simulink model "PMSM_vector_control_sim"  (R2019a)
settings: Solver=ode4  StartTime=0.0  StopTime=Tfinal  FixedStep=Ts  RelTol=1e-3  EnableMultiTasking=on
values from neighbouring files (symbols this model uses):
  Cdc = 150e-6    (= 0.00015)    [PMSM_modular_vector_control_sim_parameters.m]    (also in PMSM_vector_control_single_parameters.m)
  EfRated = 80    [PMSM_modular_vector_control_sim_parameters.m]    (also in PMSM_vector_control_single_parameters.m)
  fout = 100    [PMSM_modular_vector_control_sim_parameters.m]    (also in PMSM_vector_control_single_parameters.m)
  IdPIDmax = Vdcm/5    (= 20)    [PMSM_modular_vector_control_sim_parameters.m]    (also in PMSM_vector_control_single_parameters.m = 54)
  IdPIDmin = -Vdcm/5    (= -20)    [PMSM_modular_vector_control_sim_parameters.m]    (also in PMSM_vector_control_single_parameters.m = -54)
  Idref = 0    [PMSM_vector_control_single_parameters.m]
  Inertia = 1e-2    (= 0.01)    [PMSM_modular_vector_control_sim_parameters.m]    (also in PMSM_vector_control_single_parameters.m)
  IqPIDmax = Vdcm-10    (= 90)    [PMSM_modular_vector_control_sim_parameters.m]    (also in PMSM_vector_control_single_parameters.m = 260)
  IqPIDmin = -(Vdcm-10)    (= -90)    [PMSM_modular_vector_control_sim_parameters.m]    (also in PMSM_vector_control_single_parameters.m = -260)
  IrefOverTref = MotorSpeedRad/(EfRated*3)    (= 0.261799387799)    [PMSM_modular_vector_control_sim_parameters.m]    (also in PMSM_vector_control_single_parameters.m)
  LoadTorque1 = 2    [PMSM_modular_vector_control_sim_parameters.m]    (also in PMSM_vector_control_single_parameters.m = 30)
  LoadTorque2 = 2    [PMSM_modular_vector_control_sim_parameters.m]    (also in PMSM_vector_control_single_parameters.m = 20)
  LoadTorqueStepTime = 3    [PMSM_modular_vector_control_sim_parameters.m]    (also in PMSM_vector_control_single_parameters.m = 0.5)
  Ls = 3.51e-3    (= 0.00351)    [PMSM_modular_vector_control_sim_parameters.m]    (also in PMSM_vector_control_single_parameters.m)
  modulation_type = 1    [PMSM_modular_vector_control_sim_parameters.m]    (also in PMSM_vector_control_single_parameters.m)
  phase = [0 0 0 0]    [PMSM_modular_vector_control_sim_parameters.m]    (also in PMSM_vector_control_single_parameters.m)
  PolePairs = 10    [PMSM_modular_vector_control_sim_parameters.m]    (also in PMSM_vector_control_single_parameters.m)
  Rin = 1e-3    (= 0.001)    [PMSM_modular_vector_control_sim_parameters.m]    (also in PMSM_vector_control_single_parameters.m)
  Ripth = 0.1    [PMSM_modular_vector_control_sim_parameters.m]    (also in PMSM_vector_control_single_parameters.m)
  Rs = 321e-3    (= 0.321)    [PMSM_modular_vector_control_sim_parameters.m]    (also in PMSM_vector_control_single_parameters.m)
  SpeedPIDmax = 20    [PMSM_modular_vector_control_sim_parameters.m]    (also in PMSM_vector_control_single_parameters.m = 60)
  SpeedPIDmin = -20    [PMSM_modular_vector_control_sim_parameters.m]    (also in PMSM_vector_control_single_parameters.m = -60)
  SpeedRef1 = 200    [PMSM_modular_vector_control_sim_parameters.m]    (also in PMSM_vector_control_single_parameters.m = 600)
  SpeedRef2 = 100    [PMSM_modular_vector_control_sim_parameters.m]    (also in PMSM_vector_control_single_parameters.m = 200)
  SpeedRefStepTime = 6    [PMSM_modular_vector_control_sim_parameters.m]    (also in PMSM_vector_control_single_parameters.m = 0.5)
  Ts = 1000e-9    (= 1e-06)    [PMSM_modular_vector_control_sim_parameters.m]    (also in PMSM_vector_control_single_parameters.m)
  Vdc = 200    [PMSM_modular_vector_control_sim_parameters.m]    (also in PMSM_vector_control_single_parameters.m = 270)
  Vin = Vdc + Rin*(Pout/Vdc)    (= 200.01)    [PMSM_modular_vector_control_sim_parameters.m]    (also in PMSM_vector_control_single_parameters.m = 270.007407407)
  ViscousFriction = 1e-3    (= 0.001)    [PMSM_modular_vector_control_sim_parameters.m]    (also in PMSM_vector_control_single_parameters.m)
undefined symbols (not defined in the file or in its folder): delta, Lload, ma, Rload
libraries: powerlib x28, powerlib_meascontrol x25, simulink x6, electricdrivelib x1
settings Model: Creator=ugurm  LastModifiedBy=hakan
settings DataIOCC: LimitDataPoints=on  SaveFormat=Array  ReturnWorkspaceOutputs=off
settings OptimizationCC: LifeSpan=inf
settings DebuggingCC: UnderspecifiedInitializationDetection=Classic  MergeDetectMultiDrivingBlocksExec=none  SolverPrmCheckMsg=warning  StateNameClashWarn=warning  SFUnexpectedBacktrackingDiag=warning  SFNoUnconditionalDefaultTransitionDiag=warning  ArithmeticOperatorsInVariantConditions=warning
settings HardwareCC: ProdBitPerPointer=32  ProdBitPerSizeT=32  ProdBitPerPtrDiffT=32  ProdLargestAtomicFloat=None  ProdIntDivRoundTo=Undefined  ProdEndianess=Unspecified  ProdWordSize=32  ProdHWDeviceType=32-bit Generic
settings ModelReferenceCC: PropagateSignalLabelsOutOfModel=off
settings SFSimCC: SimUseLocalCustomCode=off
settings RTWCC: RTWUseLocalCustomCode=off
settings CodeAppCC: StateflowObjectComments=on
settings GRTTargetCC: TargetLangStandard=C89/C90 (ANSI)  GeneratePreprocessorConditionals=Disable all
settings ConfigComp: CovMetricSettings=dw  CovHtmlReporting=on  CovSaveCumulativeToWorkspaceVar=on  CovSaveSingleToWorkspaceVar=on  CovExternalEMLEnable=off
settings SimscapeCC: SimscapeNormalizeSystem=off

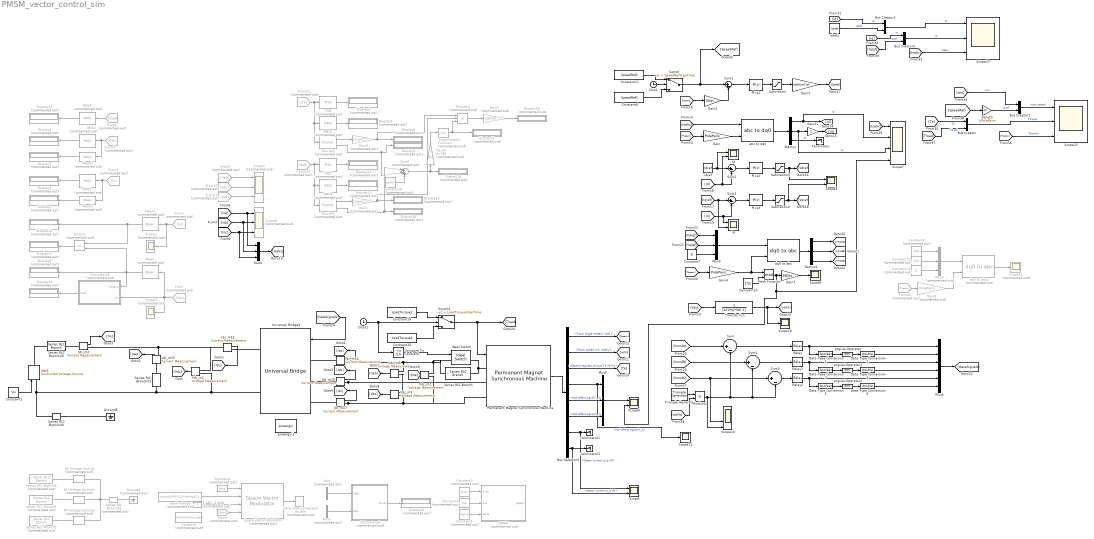
== system PMSM_vector_control_sim ==
  "1:ABC, -1:ACB" : Constant  Commented=on  Value=-1
  AC Voltage Source : powerlib/Electrical Sources/AC Voltage Source  Commented=on  Amplitude=EfRated*sqrt(2)  Phase=0  Frequency=fout  SampleTime=0  Measurements=None  BusType=swing  Pref=10e3  Qref=0  Qmin=-inf  Qmax=+inf
      settings: SourceProductName=Simscape Electrical
  AC Voltage Source1 : powerlib/Electrical Sources/AC Voltage Source  Commented=on  Amplitude=EfRated*sqrt(2)  Phase=-120  Frequency=fout  SampleTime=0  Measurements=None  BusType=swing  Pref=10e3  Qref=0  Qmin=-inf  Qmax=+inf
      settings: SourceProductName=Simscape Electrical
  AC Voltage Source2 : powerlib/Electrical Sources/AC Voltage Source  Commented=on  Amplitude=EfRated*sqrt(2)  Phase=120  Frequency=fout  SampleTime=0  Measurements=None  BusType=swing  Pref=10e3  Qref=0  Qmin=-inf  Qmax=+inf
      settings: SourceProductName=Simscape Electrical
  Bus Creator{,1..3} (4 alike) : BusCreator  Inputs=2
  Bus Selector3 : BusSelector  OutputSignals=Rotor angle thetam (rad),Rotor speed wm (rad/s),Electromagnetic torque Te (N*m),Hall effect signal h_a,Hall effect signal h_b,Hall effect signal h_c,Stator current is_q (A),Stator current is_d (A)
  Clock : Clock
  Clock1 : Clock
  Compare To Constant : simulink/Logic and Bit Operations/Compare To Constant  relop=<=  const=3.0  OutDataTypeStr=boolean
  Constant : Constant  Commented=on  Value=modulation_type
  Constant1 : Constant  Value=Vin
  Constant10 : Constant  Value=2*pi
  Constant11 : Constant  Value=SpeedRef2
  Constant12 : Constant  Commented=on  Value=100
  Constant13 : Constant  Commented=on  Value=0
  Constant14 : Constant  Value=LoadTorque2
  Constant15 : Constant  Value=LoadTorque1
  Constant2 : Constant  Commented=on  Value=fout
  Constant3 : Constant  Commented=on  Value=fout
  Constant4 : Constant  Commented=on  Value=ma
  Constant5 : Constant  Commented=on  Value=delta
  Constant6 : Constant  Value=SpeedRef1
  Constant7 : Constant  Value=0
  Constant8 : Constant  Commented=on  Value=100
  Constant9 : Constant  Commented=on  Value=sqrt(3)
  Data Type Conversion : DataTypeConversion  Commented=on  OutDataTypeStr=double
  Data Type Conversion1 : DataTypeConversion  OutDataTypeStr=boolean
  Data Type Conversion2 : DataTypeConversion  OutDataTypeStr=double
  Data Type Conversion3 : DataTypeConversion  OutDataTypeStr=boolean
  Data Type Conversion4 : DataTypeConversion  OutDataTypeStr=double
  Data Type Conversion5 : DataTypeConversion  OutDataTypeStr=boolean
  Data Type Conversion6 : DataTypeConversion  OutDataTypeStr=double
  Demux : Demux  Outputs=3
  Demux1 : Demux  Outputs=3
  Display{1..21} (21 alike) : Display  Commented=on
  Fourier1 : powerlib_meascontrol/Measurements/Fourier  Commented=on  Freq=fout  n=1  InInit=[0, 0]  Ts=Ts
      settings: SourceProductName=Simscape Electrical
  Fourier2 : powerlib_meascontrol/Measurements/Fourier  Commented=on  Freq=fout  n=1  InInit=[0, 0]  Ts=Ts
      settings: SourceProductName=Simscape Electrical
  From : From  Commented=on  GotoTag=Vdc
  From1 : From  Commented=on  GotoTag=Iin
  From10 : From  Commented=on  GotoTag=Vbc
  From11 : From  Commented=on  GotoTag=Vca
  From12 : From  Commented=on  GotoTag=Isa
  From15 : From  Commented=on  GotoTag=Vab
  From2 : From  Commented=on  GotoTag=Iin
  From3 : From  Commented=on  GotoTag=Idc
  From30 : From  Commented=on  GotoTag=Thetam
  From4 : From  Commented=on  GotoTag=Icap
  From5 : From  Commented=on  GotoTag=Vdc
  From9 : From  Commented=on  GotoTag=Vab
  Gain : Gain  Gain=PolePairs
  Gain1 : Gain  Commented=on  Gain=1/sqrt(2)
  Gain10 : Gain  Gain=1/PolePairs
  Gain11 : Gain
  Gain2 : Gain  Gain=30/pi
  Gain3 : Gain  Gain=IrefOverTref
  Gain4 : Gain  Gain=PolePairs
  Gain5 : Gain  Commented=on  Gain=sqrt(3)
  Gain6 : Gain  Commented=on  Gain=pi/180
  Gain7 : Gain  Gain=180/pi
  Gain8 : Gain  Commented=on  Gain=PolePairs
  Gain9 : Gain  Commented=on  Gain=1/sqrt(2)
  Ground5 : powerlib/Elements/Ground  LConnTagsString=a
      settings: SourceProductName=Simscape Electrical
  Ground6 : powerlib/Elements/Ground  Commented=on  LConnTagsString=a
      settings: SourceProductName=Simscape Electrical
  Id : Scope  NumInputPorts=2
  Idc_m{2,11,14..17} (6 alike) : powerlib/Measurements/Current Measurement  PhasorSimulation=off  OutputType=Complex  PSBequivalent=0
      settings: SourceProductName=Simscape Electrical
  Ideal Switch : powerlib/Power Electronics/Ideal Switch  Ron=0.001  Lon=0  IC=0  Rs=1e5  Cs=inf  Measurements=on
      settings: SourceProductName=Simscape Electrical
  Iq : Scope  NumInputPorts=2
  Logical Operator : Logic  Operator=NOT  AllPortsSameDT=off  OutDataTypeStr=boolean
  Logical Operator1 : Logic  Operator=NOT  AllPortsSameDT=off  OutDataTypeStr=boolean
  Logical Operator2 : Logic  Operator=NOT  AllPortsSameDT=off  OutDataTypeStr=boolean
  Math Function : Math  Operator=mod  SaturateOnIntegerOverflow=on
  Mean{,1..3} (4 alike) : powerlib_meascontrol/Measurements/Mean  Commented=on  Freq=fout  Vinit=0  Ts=0
      settings: SourceProductName=Simscape Electrical
  Mux : Mux  Commented=on  Inputs=3
  Mux1 : Mux  Commented=on  Inputs=3
  Mux2 : Mux  Inputs=3
  Mux3 : Mux  Inputs=3
  Mux4 : Mux  Inputs=6
  Mux5 : Mux  Inputs=3
  Mux6 : Mux  Commented=on  Inputs=3
  PI iq1 : simulink/Continuous/PID Controller  Controller=PI  Form=Parallel  TimeDomain=Discrete-time  SampleTime=-1  IntegratorMethod=Forward Euler  FilterMethod=Forward Euler  ControllerParametersSource=internal  P=0.1  I=1  D=0  UseFilter=on  N=100  TunerSelectOption=Transfer Function Based (PID Tuner App)  InitialConditionSource=internal  InitialConditionForIntegrator=0  InitialConditionForFilter=0  DifferentiatorICPrevScaledInput=0  ExternalReset=none  TrackingMode=off  Kt=1  LimitOutput=off  UpperSaturationLimit=inf  LowerSaturationLimit=-inf  LinearizeAsGain=on  AntiWindupMode=none  Kb=1  POutMin=[]  POutMax=[]  IOutMin=[]  IOutMax=[]  DOutMin=[]  DOutMax=[]  NOutMin=[]  NOutMax=[]  SumOutMin=[]  SumOutMax=[]  SaturationOutMin=[]  SaturationOutMax=[]  PParamMin=[]  PParamMax=[]  IParamMin=[]  IParamMax=[]  DParamMin=[]  DParamMax=[]  NParamMin=[]  NParamMax=[]  KbParamMin=[]  KbParamMax=[]  KtParamMin=[]  KtParamMax=[]  KbOutMin=[]  KbOutMax=[]  KtOutMin=[]  KtOutMax=[]  IntegratorOutMin=[]  IntegratorOutMax=[]  FilterOutMin=[]  FilterOutMax=[]  SumI1OutMin=[]  SumI1OutMax=[]  SumI2OutMin=[]  SumI2OutMax=[]  SumI3OutMin=[]  SumI3OutMax=[]  SumI4OutMin=[]  SumI4OutMax=[]  SumDOutMin=[]  SumDOutMax=[]  DifferentiatorOutMin=[]  DifferentiatorOutMax=[]  FilterDiffOutCoefMin=[]  FilterDiffOutCoefMax=[]  ReciprocalOutMin=[]  ReciprocalOutMax=[]  SumDenOutMin=[]  SumDenOutMax=[]  SumNumOutMin=[]  SumNumOutMax=[]  DivideOutMin=[]  DivideOutMax=[]  IntegratorContinuousStateAttributes=''  IntegratorStateMustResolveToSignalObject=off  IntegratorRTWStateStorageClass=Auto  FilterContinuousStateAttributes=''  FilterStateMustResolveToSignalObject=off  FilterRTWStateStorageClass=Auto  ParallelPVariant=InternalParameters  IdealPVariant=Disabled  IVariant=InternalParameters  DVariant=Disabled  IntegratorVariant=Discrete  SatVariant=Disabled  AWVariant=Passthrough  PCopyVariant=Disabled  TRVariant=Disabled  FdbkBlocksVariant=Forward  IdealPFdbkVariant=Disabled  SatFdbkVariant=Disabled  DerivativeFilterVariant=Disabled  NVariant=Disabled  NCopyVariant=Disabled_SignalSpec  FilterICVariant=Disabled  IntegratorICVariant=InternalICs  ExternalResetVariant=Disabled  TRSumVariant=Passthrough  SumFdbkVariant=Disabled  SumVariant=Sum_PI
  PI iq2 : simulink/Continuous/PID Controller  Controller=PI  Form=Parallel  TimeDomain=Discrete-time  SampleTime=-1  IntegratorMethod=Forward Euler  FilterMethod=Forward Euler  ControllerParametersSource=internal  P=100  I=100  D=0  UseFilter=on  N=100  TunerSelectOption=Transfer Function Based (PID Tuner App)  InitialConditionSource=internal  InitialConditionForIntegrator=0  InitialConditionForFilter=0  DifferentiatorICPrevScaledInput=0  ExternalReset=none  TrackingMode=off  Kt=1  LimitOutput=off  UpperSaturationLimit=inf  LowerSaturationLimit=-inf  LinearizeAsGain=on  AntiWindupMode=none  Kb=1  POutMin=[]  POutMax=[]  IOutMin=[]  IOutMax=[]  DOutMin=[]  DOutMax=[]  NOutMin=[]  NOutMax=[]  SumOutMin=[]  SumOutMax=[]  SaturationOutMin=[]  SaturationOutMax=[]  PParamMin=[]  PParamMax=[]  IParamMin=[]  IParamMax=[]  DParamMin=[]  DParamMax=[]  NParamMin=[]  NParamMax=[]  KbParamMin=[]  KbParamMax=[]  KtParamMin=[]  KtParamMax=[]  KbOutMin=[]  KbOutMax=[]  KtOutMin=[]  KtOutMax=[]  IntegratorOutMin=[]  IntegratorOutMax=[]  FilterOutMin=[]  FilterOutMax=[]  SumI1OutMin=[]  SumI1OutMax=[]  SumI2OutMin=[]  SumI2OutMax=[]  SumI3OutMin=[]  SumI3OutMax=[]  SumI4OutMin=[]  SumI4OutMax=[]  SumDOutMin=[]  SumDOutMax=[]  DifferentiatorOutMin=[]  DifferentiatorOutMax=[]  FilterDiffOutCoefMin=[]  FilterDiffOutCoefMax=[]  ReciprocalOutMin=[]  ReciprocalOutMax=[]  SumDenOutMin=[]  SumDenOutMax=[]  SumNumOutMin=[]  SumNumOutMax=[]  DivideOutMin=[]  DivideOutMax=[]  IntegratorContinuousStateAttributes=''  IntegratorStateMustResolveToSignalObject=off  IntegratorRTWStateStorageClass=Auto  FilterContinuousStateAttributes=''  FilterStateMustResolveToSignalObject=off  FilterRTWStateStorageClass=Auto  ParallelPVariant=InternalParameters  IdealPVariant=Disabled  IVariant=InternalParameters  DVariant=Disabled  IntegratorVariant=Discrete  SatVariant=Disabled  AWVariant=Passthrough  PCopyVariant=Disabled  TRVariant=Disabled  FdbkBlocksVariant=Forward  IdealPFdbkVariant=Disabled  SatFdbkVariant=Disabled  DerivativeFilterVariant=Disabled  NVariant=Disabled  NCopyVariant=Disabled_SignalSpec  FilterICVariant=Disabled  IntegratorICVariant=InternalICs  ExternalResetVariant=Disabled  TRSumVariant=Passthrough  SumFdbkVariant=Disabled  SumVariant=Sum_PI
  PI iq3 : simulink/Continuous/PID Controller  Controller=PI  Form=Parallel  TimeDomain=Discrete-time  SampleTime=-1  IntegratorMethod=Forward Euler  FilterMethod=Forward Euler  ControllerParametersSource=internal  P=100  I=100  D=0  UseFilter=on  N=100  TunerSelectOption=Transfer Function Based (PID Tuner App)  InitialConditionSource=internal  InitialConditionForIntegrator=0  InitialConditionForFilter=0  DifferentiatorICPrevScaledInput=0  ExternalReset=none  TrackingMode=off  Kt=1  LimitOutput=off  UpperSaturationLimit=inf  LowerSaturationLimit=-inf  LinearizeAsGain=on  AntiWindupMode=none  Kb=1  POutMin=[]  POutMax=[]  IOutMin=[]  IOutMax=[]  DOutMin=[]  DOutMax=[]  NOutMin=[]  NOutMax=[]  SumOutMin=[]  SumOutMax=[]  SaturationOutMin=[]  SaturationOutMax=[]  PParamMin=[]  PParamMax=[]  IParamMin=[]  IParamMax=[]  DParamMin=[]  DParamMax=[]  NParamMin=[]  NParamMax=[]  KbParamMin=[]  KbParamMax=[]  KtParamMin=[]  KtParamMax=[]  KbOutMin=[]  KbOutMax=[]  KtOutMin=[]  KtOutMax=[]  IntegratorOutMin=[]  IntegratorOutMax=[]  FilterOutMin=[]  FilterOutMax=[]  SumI1OutMin=[]  SumI1OutMax=[]  SumI2OutMin=[]  SumI2OutMax=[]  SumI3OutMin=[]  SumI3OutMax=[]  SumI4OutMin=[]  SumI4OutMax=[]  SumDOutMin=[]  SumDOutMax=[]  DifferentiatorOutMin=[]  DifferentiatorOutMax=[]  FilterDiffOutCoefMin=[]  FilterDiffOutCoefMax=[]  ReciprocalOutMin=[]  ReciprocalOutMax=[]  SumDenOutMin=[]  SumDenOutMax=[]  SumNumOutMin=[]  SumNumOutMax=[]  DivideOutMin=[]  DivideOutMax=[]  IntegratorContinuousStateAttributes=''  IntegratorStateMustResolveToSignalObject=off  IntegratorRTWStateStorageClass=Auto  FilterContinuousStateAttributes=''  FilterStateMustResolveToSignalObject=off  FilterRTWStateStorageClass=Auto  ParallelPVariant=InternalParameters  IdealPVariant=Disabled  IVariant=InternalParameters  DVariant=Disabled  IntegratorVariant=Discrete  SatVariant=Disabled  AWVariant=Passthrough  PCopyVariant=Disabled  TRVariant=Disabled  FdbkBlocksVariant=Forward  IdealPFdbkVariant=Disabled  SatFdbkVariant=Disabled  DerivativeFilterVariant=Disabled  NVariant=Disabled  NCopyVariant=Disabled_SignalSpec  FilterICVariant=Disabled  IntegratorICVariant=InternalICs  ExternalResetVariant=Disabled  TRSumVariant=Passthrough  SumFdbkVariant=Disabled  SumVariant=Sum_PI
  Permanent Magnet Synchronous Machine : powerlib/Machines/Permanent Magnet Synchronous Machine  NbPhases=3  FluxDistribution=Sinusoidal  RotorType=Round  MechanicalLoad=Torque Tm  PresetModel=No  ShowDetailedParameters=on  MeasurementBus=off  Resistance=Rs  Inductance=8.5e-3  dqInductances=[3.1e-3,3.6e-3]  La=Ls  MachineConstant=Voltage Constant (V_peak L-L / krpm)  Flux=0.18006  VoltageCst=VoltageConstant  TorqueCst=2.7009  Flat=120  Mechanical=[Inertia ViscousFriction PolePairs 0]  PolePairs=4  InitialConditions=[0,0, 0,0]  InitialConditions5ph=[0 0 0 0 0 0]  TsPowergui=0  TsBlock=-1  RefAngle=90 degrees behind phase A axis (modified Park)
  Product : Product  Commented=on
  Product1 : Product
  Product2 : Product  Commented=on  Inputs=3
  RMS{1..5} (5 alike) : powerlib_meascontrol/Measurements/RMS  Commented=on  TrueRMS=on  Freq=fout  RMSInit=0  Ts=0
      settings: SourceProductName=Simscape Electrical
  Relay : Relay
  Relay1 : Relay
  Relay2 : Relay
  SPWM : Subsystem  Commented=on
  Saturation : Saturate  UpperLimit=SpeedPIDmax  LowerLimit=SpeedPIDmin
  Saturation1 : Saturate  UpperLimit=IdPIDmax  LowerLimit=IdPIDmin
  Saturation2 : Saturate  UpperLimit=IqPIDmax  LowerLimit=IqPIDmin
  Scope : Scope  NumInputPorts=2
  Scope1 : Scope  Commented=on
  Scope10 : Scope  NumInputPorts=4
  Scope11 : Scope
  Scope12 : Scope  Commented=on
  Scope13 : Scope  NumInputPorts=3
  Scope15 : Scope  NumInputPorts=3
  Scope16 : Scope
  Scope2 : Scope  Commented=on  NumInputPorts=3
  Scope3 : Scope  Commented=on
  Scope5 : Scope  NumInputPorts=2
  Scope6 : Scope
  Scope7 : Scope  NumInputPorts=4
  Scope8 : Scope  Commented=on  NumInputPorts=3
  Scope9 : Scope  NumInputPorts=2
  Series RLC Branch : powerlib/Elements/Series RLC Branch  LConnTagsString=__new0  RConnTagsString=__new0  BranchType=R  Resistance=5000  Inductance=1e-3  SetiL0=off  InitialCurrent=0  Capacitance=1e-6  Setx0=off  InitialVoltage=0  Measurements=None
      settings: SourceProductName=Simscape Electrical
  Series RLC Branch1 : powerlib/Elements/Series RLC Branch  Commented=on  LConnTagsString=__new0  RConnTagsString=__new0  BranchType=RL  Resistance=Rs  Inductance=Ls  SetiL0=off  InitialCurrent=0  Capacitance=1e-6  Setx0=off  InitialVoltage=0  Measurements=None
      settings: SourceProductName=Simscape Electrical
  Series RLC Branch2 : powerlib/Elements/Series RLC Branch  Commented=on  LConnTagsString=__new0  RConnTagsString=__new0  BranchType=RL  Resistance=Rs  Inductance=Ls  SetiL0=off  InitialCurrent=0  Capacitance=1e-6  Setx0=off  InitialVoltage=0  Measurements=None
      settings: SourceProductName=Simscape Electrical
  Series RLC Branch20 : powerlib/Elements/Series RLC Branch  LConnTagsString=__new0  RConnTagsString=__new0  BranchType=R  Resistance=Rin  Inductance=1e-3  SetiL0=off  InitialCurrent=0  Capacitance=1e-6  Setx0=off  InitialVoltage=0  Measurements=None
      settings: SourceProductName=Simscape Electrical
  Series RLC Branch21 : powerlib/Elements/Series RLC Branch  LConnTagsString=__new0  RConnTagsString=__new0  BranchType=C  Resistance=Rload  Inductance=Lload  SetiL0=off  InitialCurrent=0  Capacitance=Cdc  Setx0=off  InitialVoltage=0  Measurements=None
      settings: SourceProductName=Simscape Electrical
  Series RLC Branch40 : powerlib/Elements/Series RLC Branch  LConnTagsString=__new0  RConnTagsString=__new0  BranchType=R  Resistance=1e12  Inductance=Lload  SetiL0=off  InitialCurrent=0  Capacitance=1e-6  Setx0=off  InitialVoltage=0  Measurements=None
      settings: SourceProductName=Simscape Electrical
  Series RLC Branch42 : powerlib/Elements/Series RLC Branch  Commented=on  LConnTagsString=__new0  RConnTagsString=__new0  BranchType=R  Resistance=1e12  Inductance=Lload  SetiL0=off  InitialCurrent=0  Capacitance=1e-6  Setx0=off  InitialVoltage=0  Measurements=None
      settings: SourceProductName=Simscape Electrical
  Series RLC Branch6 : powerlib/Elements/Series RLC Branch  Commented=on  LConnTagsString=__new0  RConnTagsString=__new0  BranchType=RL  Resistance=Rs  Inductance=Ls  SetiL0=off  InitialCurrent=0  Capacitance=1e-6  Setx0=off  InitialVoltage=0  Measurements=None
      settings: SourceProductName=Simscape Electrical
  Space Vector Modulator : electricdrivelib/Fundamental Drive Blocks/Space Vector Modulator  Commented=on  LabelModeActiveChoice=Detailed  detailLevel=Detailed  fc_bus=50  car_freq=fsw  TsMLIV=1e-6  Ts=Ts
      settings: AttributesFormatString=%<BlockChoice>  SourceProductName=Simscape Electrical  SourceProductBaseCode=PS
  Subsystem4 : Subsystem  Commented=on
  Subsystem5 : Subsystem  Commented=on
  Sum{,1..5} (6 alike) : Sum  Inputs=|+-
  Sum6 : Sum  Commented=on  Inputs=|+--
  Switch : Switch  Criteria=u2 > Threshold  Threshold=SpeedRefStepTime
  Switch1 : Switch  Criteria=u2 > Threshold  Threshold=LoadTorqueStepTime
  THD : powerlib_meascontrol/Measurements/THD  Commented=on  Freq=50  Ts=0
      settings: SourceProductName=Simscape Electrical
  THD1 : powerlib_meascontrol/Measurements/THD  Commented=on  Freq=50  Ts=0
      settings: SourceProductName=Simscape Electrical
  Terminator : Terminator
  Terminator1 : Terminator
  Terminator2 : Terminator
  Transfer Fcn : TransferFcn  Denominator=[1/(2*pi*50) 1]
  Triangle Generator : powerlib_meascontrol/Pulse & Signal Generators/Triangle Generator  Freq=fsw  Phase=phase(1)  Ts=Ts
      settings: SourceProductName=Simscape Electrical
  Trigonometric Function : Trigonometry  Commented=on  Operator=cos
  Universal Bridge4 : powerlib/Power Electronics/Universal Bridge  Arms=3  SnubberResistance=1e5  SnubberCapacitance=inf  Device=IGBT / Diodes  Ron=1e-6  Lon=0  ForwardVoltages="[  0  0  ]"  ForwardVoltage=0  GTOparameters=[ 10e-6 , 20e-6 ]  IGBTparameters=[0,0]  Measurements=None  Measurements_2=None  converterType=Rectifier
      settings: SourceProductName=Simscape Electrical
  Vdc1 : powerlib/Electrical Sources/Controlled Voltage Source  Initialize=off  Source_Type=DC  Amplitude=200  Phase=0  Frequency=0  Measurements=None
      settings: SourceProductName=Simscape Electrical
  Vdc_m{1..3,5} (4 alike) : powerlib/Measurements/Voltage Measurement  PhasorSimulation=off  OutputType=Complex  PSBequivalent=0
      settings: SourceProductName=Simscape Electrical
  abc to dq0 : powerlib_meascontrol/Transformations/abc to dq0  Alignment=90 degrees behind phase A axis
      settings: SourceProductName=Simscape Electrical
  dq0 to abc : powerlib_meascontrol/Transformations/dq0 to abc  Alignment=90 degrees behind phase A axis
      settings: SourceProductName=Simscape Electrical
  dq0 to abc1 : powerlib_meascontrol/Transformations/dq0 to abc  Commented=on  Alignment=Aligned with phase A axis
      settings: SourceProductName=Simscape Electrical
  idref : Constant  Value=Idref
  idref1 : Constant  Value=Idref
  peak voltage : Constant  Commented=on  Value=ma/sqrt(3)*0.612*Vdc*sqrt(2)
  powergui1 : powerlib/powergui  Priority=1  SimulationMode=Discrete  SampleTime=Ts  frequency=60  Iterations=50  frequencyindice=0  Pbase=100e6  ErrMax=1e-4  UnitsV=kV  UnitsW=MW  buscounter=0  FunctionMessages=off  echomessages=off  EnableUseOfTLC=off  CurrentSourceSwitches=off  DisableSnubberDevices=off  DisableRonSwitches=off  DisableVfSwitches=off  DisplayEquations=off  AutomaticDiscreteSolvers=off  SolverType=Tustin  Interpol=off  ExternalGateDelay=off  methode=off  Ts=0  x0status=blocks  SPID=off  SwTol=0  HookPort=off  NonlinearTolerance=0  nMaxIteration=15  ContinueOnMaxIteration=off  RestoreLinks=warning  ResistiveCurrentMeasurement=off  Frange=[0:2:500]  Ylog=off  Xlog=on  ShowGrid=off  save=off  variable=ZData  structure=Icap  ZoomFFT=off  StartTime=0.04  cycles=5  DisplayStyle=3  fundamental=150  FreqAxis=off  MaxFrequency=1000  frequencyindicesteady=1  RmsSteady=1  display=off
      settings: SourceProductName=Simscape Electrical
  wires:
  Idc_m14/1 -> [Isa]
  Constant1/1 -> Vdc1/1
  Idc_m15/1 -> [Icap]
  Idc_m16/1 -> [Isb]
  Idc_m17/1 -> [Isc]
  Mean/1 -> Product/2, Subsystem5/1(Vdcavg), Display8/1
  RMS2/1 -> Display4/1
  Idc_m11/1 -> [Idc]
  Mean3/1 -> Display7/1
  Subsystem5/1(Out1) -> Display14/1
  Product/1 -> Display17/1
  Mux/1 -> Subsystem4/1(Vabc)
  Mux1/1 -> Subsystem4/2(Iabc)
  Subsystem4/1(Poutp) -> Display20/1
  From/1 -> Scope3/1, Mean/1, Subsystem5/2(vdc)
  Mean1/1 -> Display1/1
  RMS1/1 -> Display2/1
  Fourier1/1 -> Gain9/1
  THD/1 -> Display3/1
  RMS4/1 -> Display5/1
  Gain9/1 -> Product2/1, Display6/1
  Fourier1/2 -> Sum6/2, Display9/1
  Vdc_m1/1 -> [Vdc]
  Idc_m2/1 -> [Iin]
  Mean2/1 -> Product/1, Display10/1
  From1/1 -> Scope1/1, Mean2/1
  From2/1 -> Mean1/1, RMS1/1
  From3/1 -> Mean3/1, RMS2/1
  From4/1 -> RMS5/1
  RMS5/1 -> Display11/1
  Constant2/1 -> Space Vector Modulator/1
  From5/1 -> Space Vector Modulator/4
  "1:ABC, -1:ACB"/1 -> Space Vector Modulator/3
  peak voltage/1 -> Space Vector Modulator/2
  Vdc_m5/1 -> [Vab]
  Vdc_m3/1 -> [Vbc]
  Vdc_m2/1 -> [Vca]
  [Isa] -> Mux2/1, Scope8/1
  [Isb] -> Mux2/2, Scope8/2
  [Isc] -> Mux2/3, Scope8/3
  From9/1 -> Scope2/1
  From10/1 -> Scope2/2
  From11/1 -> Scope2/3
  From12/1 -> Fourier1/1, RMS4/1, THD/1
  THD1/1 -> Display12/1
  RMS3/1 -> Display13/1
  From15/1 -> Fourier2/1, RMS3/1, THD1/1
  Space Vector Modulator/1 -> Data Type Conversion/1
  Constant3/1 -> SPWM/1(Freq)
  Constant4/1 -> SPWM/2(ma)
  Constant5/1 -> SPWM/3(delta)
  Permanent Magnet Synchronous Machine/1 -> Bus Selector3/1
  Bus Selector3/3 -> [Te]  "<Electromagnetic torque Te (N*m)>"
  Bus Selector3/2 -> [wm]  "<Rotor speed wm (rad/s)>"
  Bus Selector3/1 -> [Thetam]  "<Rotor angle thetam (rad)>"
  Mux2/1 -> [Isabc]
  [Isabc] -> abc to dq0/1
  Gain/1 -> abc to dq0/2
  [Thetam] -> Gain/1
  abc to dq0/1 -> Demux/1
  Demux/1 -> [id], Scope7/2  "id"
  Demux/2 -> Gain11/1, Scope7/3  "iq"
  Demux/3 -> Terminator/1  "i0"
  Fourier2/1 -> Gain1/1
  Gain1/1 -> Product2/2, Display15/1
  Fourier2/2 -> Sum6/1, Display16/1
  [wm] -> Gain2/1
  Gain2/1 -> Sum1/2
  Switch/1 -> [SpeedRef], Sum1/1
  Sum1/1 -> PI iq1/1
  PI iq1/1 -> Saturation/1
  Saturation/1 -> Gain3/1
  Gain3/1 -> [Iqref]
  [id] -> Id/2, Sum2/2
  Sum2/1 -> PI iq2/1
  PI iq2/1 -> Saturation1/1
  idref/1 -> Id/1, Sum2/1
  [iq] -> Iq/1, Sum3/2
  Sum3/1 -> PI iq3/1
  PI iq3/1 -> Saturation2/1
  [Iqref] -> Iq/2, Sum3/1
  Saturation2/1 -> [Vqref], Scope9/2
  [Thetam] -> Gain4/1
  Gain4/1 -> Math Function/1, dq0 to abc/2
  Constant7/1 -> Mux3/3
  Mux3/1 -> dq0 to abc/1
  [Vdc] -> Transfer Fcn/1
  Transfer Fcn/1 -> Scope16/1, [VdcFilt]
  dq0 to abc/1 -> Demux1/1
  Sum/1 -> Relay/1
  Sum4/1 -> Relay1/1
  Sum5/1 -> Relay2/1
  Data Type Conversion1/1 -> Logical Operator/1
  Logical Operator/1 -> Data Type Conversion2/1
  Data Type Conversion2/1 -> Mux4/2
  Data Type Conversion3/1 -> Logical Operator1/1
  Relay1/1 -> Data Type Conversion3/1, Mux4/3
  Logical Operator1/1 -> Data Type Conversion4/1
  Data Type Conversion4/1 -> Mux4/4
  Data Type Conversion5/1 -> Logical Operator2/1
  Relay2/1 -> Data Type Conversion5/1, Mux4/5
  Logical Operator2/1 -> Data Type Conversion6/1
  Data Type Conversion6/1 -> Mux4/6
  Relay/1 -> Mux4/1, Data Type Conversion1/1
  [VmodC] -> Scope10/3, Sum5/1
  Triangle Generator/1 -> Product1/1
  [VdcFilt] -> Product1/2
  Demux1/1 -> [VmodA]
  Demux1/2 -> [VmodB]
  Demux1/3 -> [VmodC]
  Mux4/1 -> [GateSignals]
  Switch1/1 -> [Tload], Permanent Magnet Synchronous Machine/1
  [GateSignals] -> Universal Bridge4/1
  Product1/1 -> Scope10/4, Sum/2, Sum4/2, Sum5/2
  Constant9/1 -> Sum6/3
  Sum6/1 -> Display18/1, Gain6/1
  Trigonometric Function/1 -> Display21/1, Product2/3
  Gain6/1 -> Trigonometric Function/1
  Product2/1 -> Gain5/1
  Gain5/1 -> Display19/1
  Bus Selector3/6 -> Mux5/3  "<Hall effect signal h_c>"
  Bus Selector3/5 -> Mux5/2  "<Hall effect signal h_b>"
  Bus Selector3/4 -> Scope11/1, Mux5/1  "<Hall effect signal h_a>"
  Mux5/1 -> Scope5/1
  Constant10/1 -> Math Function/2
  Math Function/1 -> Scope7/4, Scope5/2, Gain7/1
  Gain7/1 -> Scope6/1
  [Isabc] -> Scope7/1
  Gain11/1 -> [iq]
  Bus Selector3/7 -> Scope/1, Terminator1/1  "<Stator current is_q (A)>"
  Bus Selector3/8 -> Scope/2, Terminator2/1  "<Stator current is_d (A)>"
  Saturation1/1 -> [Vdref], Scope9/1
  [Vqref] -> Mux3/2
  [Vdref] -> Mux3/1
  Clock/1 -> Switch/2
  Constant11/1 -> Switch/1
  Constant6/1 -> Switch/3
  Clock1/1 -> Compare To Constant/1, Switch1/2
  Constant14/1 -> Switch1/1
  Constant15/1 -> Switch1/3
  Mux6/1 -> dq0 to abc1/1
  Constant8/1 -> Mux6/1
  Constant12/1 -> Mux6/2
  Constant13/1 -> Mux6/3
  From30/1 -> Gain8/1
  Gain8/1 -> dq0 to abc1/2
  dq0 to abc1/1 -> Scope12/1
  [VmodA] -> Sum/1
  [VmodB] -> Sum4/1
  Bus Creator3/1 -> Scope13/2  "iq"
  [Isabc] -> Scope13/3  "isabc"
  [Thetam] -> Scope15/3  "Position"
  Compare To Constant/1 -> Ideal Switch/1
  [Te] -> Bus Creator/1  "Te"
  [Tload] -> Bus Creator/2  "Tload"
  Bus Creator/1 -> Scope15/2  "Torque"
  Bus Creator1/1 -> Scope15/1  "rotor speed"
  [wm] -> Bus Creator1/1  "wm"
  [SpeedRef] -> Gain10/1
  idref1/1 -> Bus Creator2/2  "idref"
  [id] -> Bus Creator2/1  "id"
  Bus Creator2/1 -> Scope13/1  "id"
  [iq] -> Bus Creator3/1  "iq"
  [Iqref] -> Bus Creator3/2  "iqref"
  Gain10/1 -> Bus Creator1/2  "wref"
  connections:
  Vdc_m5/LConn1 -- Series RLC Branch/LConn1 -- Ideal Switch/LConn1 -- Vdc_m2/LConn2 -- Idc_m14/RConn1
  Series RLC Branch42/RConn1 -- Ground6/LConn1
  Series RLC Branch40/RConn1 -- Ground5/LConn1
  Idc_m14/LConn1 -- Universal Bridge4/LConn1
  Idc_m15/LConn1 -- Series RLC Branch21/LConn1
  Vdc1/RConn1 -- Series RLC Branch20/LConn1
  Series RLC Branch42/LConn1 -- AC Voltage Source1/LConn1 -- AC Voltage Source2/LConn1 -- AC Voltage Source/LConn1
  Idc_m16/LConn1 -- Universal Bridge4/LConn2
  Idc_m17/LConn1 -- Universal Bridge4/LConn3
  Idc_m17/RConn1 -- Permanent Magnet Synchronous Machine/LConn3 -- Vdc_m2/LConn1 -- Vdc_m3/LConn2
  Idc_m16/RConn1 -- Permanent Magnet Synchronous Machine/LConn2 -- Vdc_m3/LConn1 -- Vdc_m5/LConn2
  Idc_m15/RConn1 -- Idc_m11/LConn1 -- Vdc_m1/LConn1 -- Idc_m2/RConn1
  Idc_m11/RConn1 -- Universal Bridge4/RConn1
  Vdc_m1/LConn2 -- Universal Bridge4/RConn2 -- Series RLC Branch21/RConn1 -- Vdc1/LConn1 -- Series RLC Branch40/LConn1
  Idc_m2/LConn1 -- Series RLC Branch20/RConn1
  AC Voltage Source/RConn1 -- Series RLC Branch6/RConn1
  Series RLC Branch1/RConn1 -- AC Voltage Source1/RConn1
  Series RLC Branch2/RConn1 -- AC Voltage Source2/RConn1
  Ideal Switch/RConn1 -- Series RLC Branch/RConn1 -- Permanent Magnet Synchronous Machine/LConn1

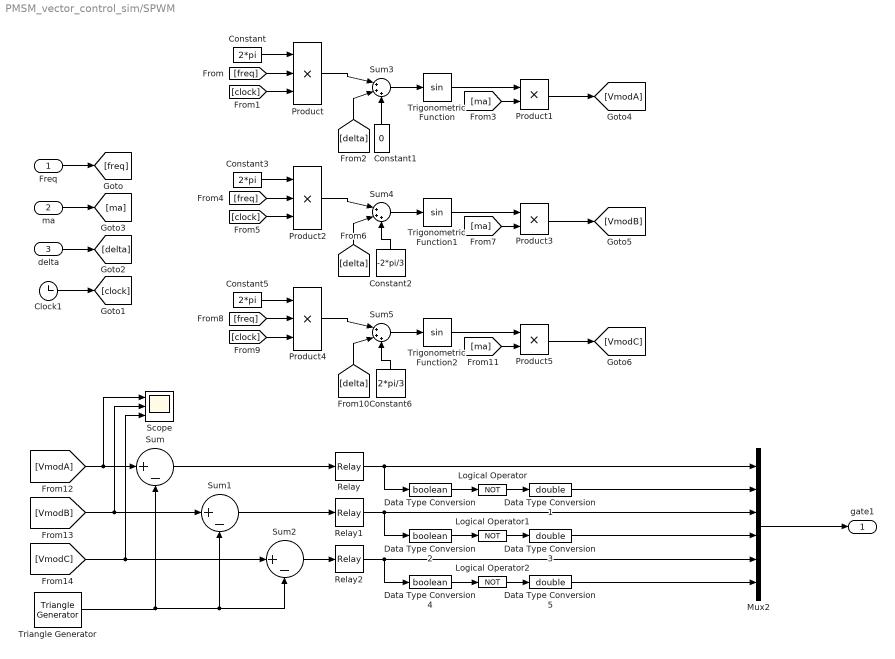
== system PMSM_vector_control_sim/SPWM ==
  Freq : Inport
  ma : Inport  Port=2
  delta : Inport  Port=3
  Clock1 : Clock
  Constant : Constant  Value=2*pi
  Constant1 : Constant  Value=0
  Constant2 : Constant  Value=-2*pi/3
  Constant3 : Constant  Value=2*pi
  Constant5 : Constant  Value=2*pi
  Constant6 : Constant  Value=2*pi/3
  Data Type Conversion : DataTypeConversion  OutDataTypeStr=boolean
  Data Type Conversion1 : DataTypeConversion  OutDataTypeStr=double
  Data Type Conversion2 : DataTypeConversion  OutDataTypeStr=boolean
  Data Type Conversion3 : DataTypeConversion  OutDataTypeStr=double
  Data Type Conversion4 : DataTypeConversion  OutDataTypeStr=boolean
  Data Type Conversion5 : DataTypeConversion  OutDataTypeStr=double
  Logical Operator : Logic  Operator=NOT  AllPortsSameDT=off  OutDataTypeStr=boolean
  Logical Operator1 : Logic  Operator=NOT  AllPortsSameDT=off  OutDataTypeStr=boolean
  Logical Operator2 : Logic  Operator=NOT  AllPortsSameDT=off  OutDataTypeStr=boolean
  Mux2 : Mux  Inputs=6
  Product : Product  Inputs=3
  Product1 : Product
  Product2 : Product  Inputs=3
  Product3 : Product
  Product4 : Product  Inputs=3
  Product5 : Product
  Relay : Relay
  Relay1 : Relay
  Relay2 : Relay
  Scope : Scope  NumInputPorts=3
  Sum : Sum  Inputs=|+-
  Sum1 : Sum  Inputs=|+-
  Sum2 : Sum  Inputs=|+-
  Sum3 : Sum  Inputs=|+++
  Sum4 : Sum  Inputs=|+++
  Sum5 : Sum  Inputs=|+++
  Triangle Generator : powerlib_meascontrol/Pulse & Signal Generators/Triangle Generator  Freq=fsw  Phase=phase(1)  Ts=Ts
      settings: SourceProductName=Simscape Electrical
  Trigonometric Function : Trigonometry
  Trigonometric Function1 : Trigonometry
  Trigonometric Function2 : Trigonometry
  gate1 : Outport
  wires:
  Triangle Generator/1 -> Sum1/2, Sum2/2, Sum/2
  [VmodB] -> Scope/2, Sum1/1
  Sum/1 -> Relay/1
  Sum1/1 -> Relay1/1
  Sum2/1 -> Relay2/1
  Data Type Conversion/1 -> Logical Operator/1
  Logical Operator/1 -> Data Type Conversion1/1
  Data Type Conversion1/1 -> Mux2/2
  Data Type Conversion2/1 -> Logical Operator1/1
  Relay1/1 -> Data Type Conversion2/1, Mux2/3
  Logical Operator1/1 -> Data Type Conversion3/1
  Data Type Conversion3/1 -> Mux2/4
  Data Type Conversion4/1 -> Logical Operator2/1
  Relay2/1 -> Data Type Conversion4/1, Mux2/5
  Logical Operator2/1 -> Data Type Conversion5/1
  Data Type Conversion5/1 -> Mux2/6
  Mux2/1 -> gate1/1
  Relay/1 -> Mux2/1, Data Type Conversion/1
  Constant/1 -> Product/1
  Product/1 -> Sum3/1
  Sum3/1 -> Trigonometric Function/1
  Trigonometric Function/1 -> Product1/1
  Freq/1 -> [freq]
  Clock1/1 -> [clock]
  [freq] -> Product/2
  [clock] -> Product/3
  [delta] -> Sum3/2
  delta/1 -> [delta]
  ma/1 -> [ma]
  [ma] -> Product1/2
  Constant1/1 -> Sum3/3
  Product1/1 -> [VmodA]
  Constant3/1 -> Product2/1
  Product2/1 -> Sum4/1
  Sum4/1 -> Trigonometric Function1/1
  Trigonometric Function1/1 -> Product3/1
  [freq] -> Product2/2
  [clock] -> Product2/3
  [delta] -> Sum4/2
  [ma] -> Product3/2
  Constant2/1 -> Sum4/3
  Product3/1 -> [VmodB]
  Constant5/1 -> Product4/1
  Product4/1 -> Sum5/1
  Sum5/1 -> Trigonometric Function2/1
  Trigonometric Function2/1 -> Product5/1
  [freq] -> Product4/2
  [clock] -> Product4/3
  [delta] -> Sum5/2
  [ma] -> Product5/2
  Constant6/1 -> Sum5/3
  Product5/1 -> [VmodC]
  [VmodA] -> Scope/1, Sum/1
  [VmodC] -> Scope/3, Sum2/1

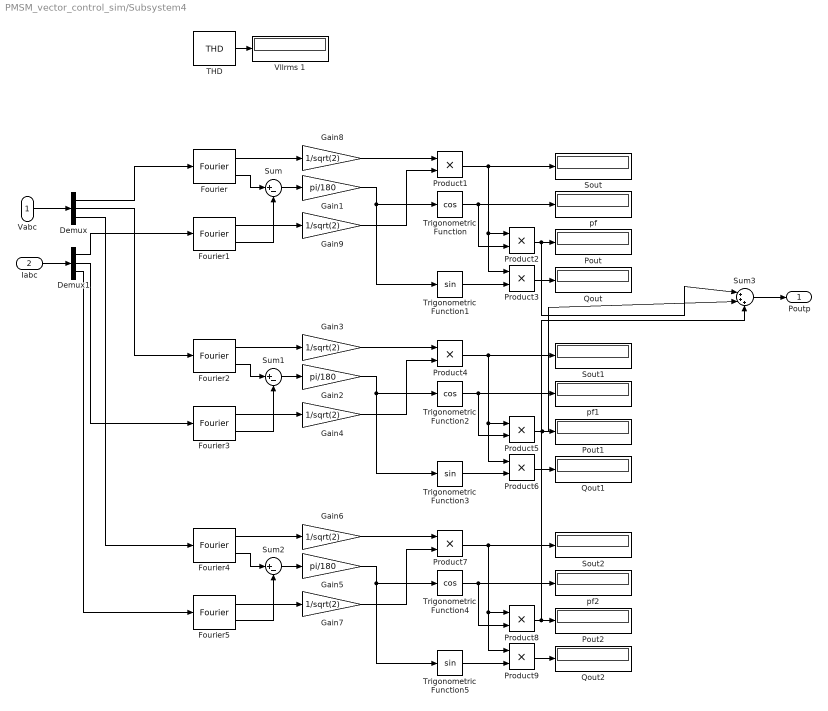
== system PMSM_vector_control_sim/Subsystem4 ==
  Vabc : Inport
  Iabc : Inport  Port=2
  Demux : Demux  Outputs=3
  Demux1 : Demux  Outputs=3
  Fourier{,1..5} (6 alike) : powerlib_meascontrol/Measurements/Fourier  Freq=fout  n=1  InInit=[0, 0]  Ts=Ts
      settings: SourceProductName=Simscape Electrical
  Gain1 : Gain  Gain=pi/180
  Gain2 : Gain  Gain=pi/180
  Gain{3..4,6..9} (6 alike) : Gain  Gain=1/sqrt(2)
  Gain5 : Gain  Gain=pi/180
  Pout : Display
  Pout1 : Display
  Pout2 : Display
  Product{1..9} (9 alike) : Product
  Qout : Display
  Qout1 : Display
  Qout2 : Display
  Sout : Display
      settings: Format=short_e
  Sout1 : Display
      settings: Format=short_e
  Sout2 : Display
      settings: Format=short_e
  Sum : Sum  Inputs=|+-
  Sum1 : Sum  Inputs=|+-
  Sum2 : Sum  Inputs=|+-
  Sum3 : Sum  Inputs=|+++
  THD : powerlib_meascontrol/Measurements/THD  Freq=fout  Ts=0
      settings: SourceProductName=Simscape Electrical
  Trigonometric Function : Trigonometry  Operator=cos
  Trigonometric Function1 : Trigonometry
  Trigonometric Function2 : Trigonometry  Operator=cos
  Trigonometric Function3 : Trigonometry
  Trigonometric Function4 : Trigonometry  Operator=cos
  Trigonometric Function5 : Trigonometry
  Vllrms 1 : Display
  pf : Display
  pf1 : Display
  pf2 : Display
  Poutp : Outport
  wires:
  Gain8/1 -> Product1/1
  Gain9/1 -> Product1/2
  Fourier1/1 -> Gain9/1
  Fourier/1 -> Gain8/1
  Product1/1 -> Product3/1, Product2/1, Sout/1
  Sum/1 -> Gain1/1
  Trigonometric Function/1 -> Product2/2, pf/1
  Gain1/1 -> Trigonometric Function1/1, Trigonometric Function/1
  Product2/1 -> Sum3/1, Pout/1
  THD/1 -> Vllrms 1/1
  Vabc/1 -> Demux/1
  Iabc/1 -> Demux1/1
  Fourier/2 -> Sum/1
  Fourier1/2 -> Sum/2
  Trigonometric Function1/1 -> Product3/2
  Product3/1 -> Qout/1
  Gain3/1 -> Product4/1
  Gain4/1 -> Product4/2
  Fourier3/1 -> Gain4/1
  Fourier2/1 -> Gain3/1
  Product4/1 -> Product6/1, Product5/1, Sout1/1
  Sum1/1 -> Gain2/1
  Trigonometric Function2/1 -> Product5/2, pf1/1
  Gain2/1 -> Trigonometric Function3/1, Trigonometric Function2/1
  Product5/1 -> Sum3/2, Pout1/1
  Fourier2/2 -> Sum1/1
  Fourier3/2 -> Sum1/2
  Trigonometric Function3/1 -> Product6/2
  Product6/1 -> Qout1/1
  Gain6/1 -> Product7/1
  Gain7/1 -> Product7/2
  Fourier5/1 -> Gain7/1
  Fourier4/1 -> Gain6/1
  Product7/1 -> Product9/1, Product8/1, Sout2/1
  Sum2/1 -> Gain5/1
  Trigonometric Function4/1 -> Product8/2, pf2/1
  Gain5/1 -> Trigonometric Function5/1, Trigonometric Function4/1
  Fourier4/2 -> Sum2/1
  Fourier5/2 -> Sum2/2
  Trigonometric Function5/1 -> Product9/2
  Product9/1 -> Qout2/1
  Product8/1 -> Sum3/3, Pout2/1
  Sum3/1 -> Poutp/1
  Demux/1 -> Fourier/1
  Demux/2 -> Fourier2/1
  Demux/3 -> Fourier4/1
  Demux1/1 -> Fourier1/1
  Demux1/2 -> Fourier3/1
  Demux1/3 -> Fourier5/1

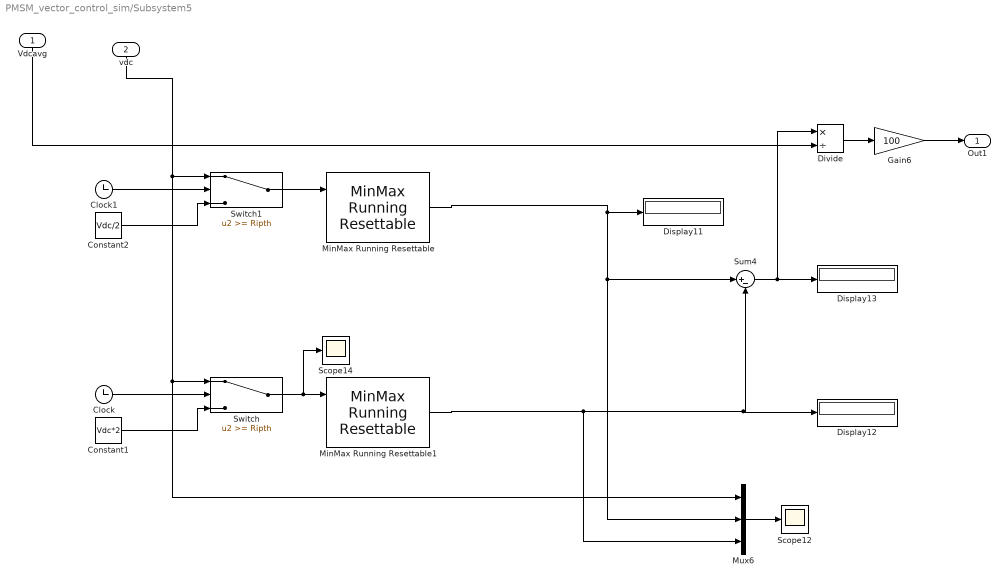
== system PMSM_vector_control_sim/Subsystem5 ==
  Vdcavg : Inport
  vdc : Inport  Port=2
  Clock : Clock
  Clock1 : Clock
  Constant1 : Constant  Value=Vdc*2  SampleTime=Ts
  Constant2 : Constant  Value=Vdc/2  SampleTime=Ts
  Display11 : Display
  Display12 : Display
  Display13 : Display
  Divide : Product  Inputs=*/
  Gain6 : Gain  Gain=100
  MinMax Running Resettable : simulink/Math Operations/MinMax Running Resettable  Function=max  vinit=0.0
  MinMax Running Resettable1 : simulink/Math Operations/MinMax Running Resettable  Function=min  vinit=Vdc*4
  Mux6 : Mux  Inputs=3
  Scope12 : Scope
  Scope14 : Scope
  Sum4 : Sum  Inputs=|+-
  Switch : Switch  Threshold=Ripth
  Switch1 : Switch  Threshold=Ripth
  Out1 : Outport
  wires:
  MinMax Running Resettable/1 -> Display11/1, Mux6/2, Sum4/1
  Clock/1 -> Switch/2
  Gain6/1 -> Out1/1
  Constant1/1 -> Switch/3
  MinMax Running Resettable1/1 -> Mux6/3, Display12/1, Sum4/2
  Switch/1 -> Scope14/1, MinMax Running Resettable1/1
  Sum4/1 -> Divide/1, Display13/1
  Divide/1 -> Gain6/1
  Mux6/1 -> Scope12/1
  Vdcavg/1 -> Divide/2
  vdc/1 -> Switch1/1, Mux6/1, Switch/1
  Switch1/1 -> MinMax Running Resettable/1
  Clock1/1 -> Switch1/2
  Constant2/1 -> Switch1/3
